simulink model "AUV_Model"  (R2019b)
settings: Solver=VariableStepAuto  StartTime=0.0  StopTime=300  FixedStep=0.5  RelTol=1e-3
InitFcn:
  | mdlWks = get_param(gcs,'ModelWorkspace');
  | a = getVariable(mdlWks,'a');
  | b = getVariable(mdlWks,'b');
  | c = getVariable(mdlWks,'c');
StopFcn:
  | figure(2)
  | plot3(Position_Data(1,1),Position_Data(1,2),Position_Data(1,3),'r*')
  | hold on
  | plot3(Position_Data(:,1),Position_Data(:,2),Position_Data(:,3));
  | plot3(Position_Data(end,1),Position_Data(end,2),Position_Data(end,3),'g*');
  | grid on
  | legend('Start Point','Trajectory','End Point')
model workspace (MAT data in the model file):
  a = 1
  b = 1
  c = 1
undefined symbols (not defined in the file or in its folder): sigbuilder_block
libraries: simulink x6, sharedtransform x6, vrlib x6, dspfdesign x6, shared6dof x1, aerolibasang x1, aerolibnav x1
(part 3 of 3)

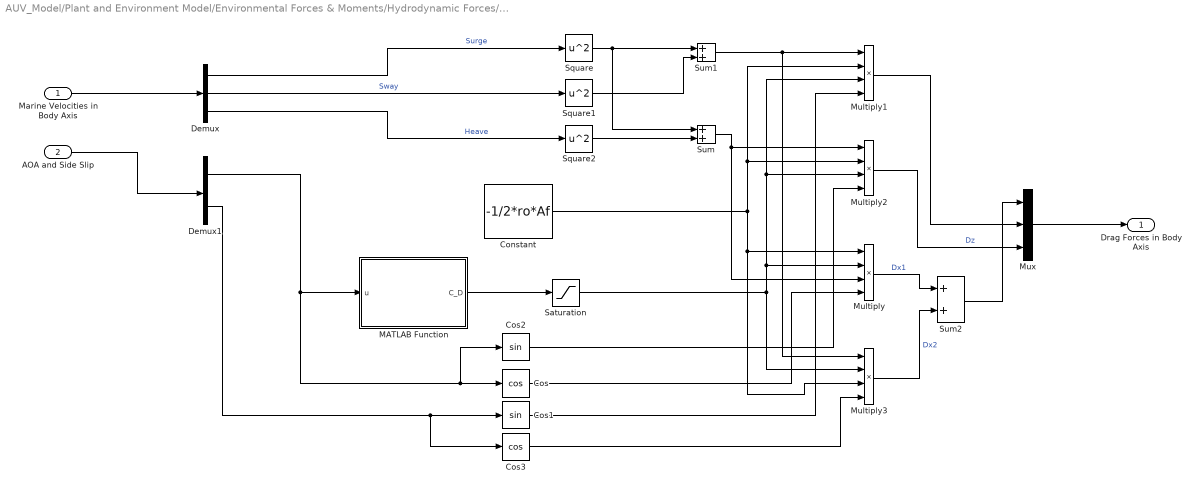
== system AUV_Model/Plant and Environment Model/Environmental Forces & Moments/Hydrodynamic Forces/Hydrodynamic Forces - Accurate/Force Exerted due to Drag (Body Axis) ==
  Marine Velocities in Body Axis : Inport
  AOA and Side Slip : Inport  Port=2
  Constant : Constant  Value=-1/2*ro*Af  mask{ro=1000, Af=0.001}
      mask prompts: ro "Density of Water"; Af "Submarine Frontal Area"
      mask DialogControl DescGroupVar Prompt: Input
      mask DialogControl DescTextVar Prompt: Enter the following values :
  Cos : Trigonometry  Operator=cos
  Cos1 : Trigonometry
  Cos2 : Trigonometry
  Cos3 : Trigonometry  Operator=cos
  Demux : Demux  Outputs=3
  Demux1 : Demux  Outputs=2
  MATLAB Function : MATLAB Function  TreatAsAtomicUnit=on
  Multiply{,1..3} (4 alike) : Product  Inputs=4
  Mux : Mux  Inputs=3
  Saturation : Saturate  UpperLimit=25  LowerLimit=-25
  Square : Math  Operator=square  SaturateOnIntegerOverflow=on
  Square1 : Math  Operator=square  SaturateOnIntegerOverflow=on
  Square2 : Math  Operator=square  SaturateOnIntegerOverflow=on
  Sum : Sum
  Sum1 : Sum
  Sum2 : Sum
  Drag Forces in Body Axis : Outport  VectorParamsAs1DForOutWhenUnconnected=off
  wires:
  Saturation/1 -> Multiply/2, Multiply2/3, Multiply1/3, Multiply3/2
  Square1/1 -> Sum1/2
  Multiply1/1 -> Mux/2
  Sum2/1 -> Mux/1
  Cos3/1 -> Multiply3/4
  AOA and Side Slip/1 -> Demux1/1
  Marine Velocities in Body Axis/1 -> Demux/1
  Cos2/1 -> Multiply2/4
  Mux/1 -> Drag Forces in Body Axis/1
  Square2/1 -> Sum/2
  Demux1/2 -> Cos1/1, Cos3/1
  Demux1/1 -> MATLAB Function/1(u), Cos2/1, Cos/1
  MATLAB Function/1(C_D) -> Saturation/1
  Multiply2/1 -> Mux/3  "Dz"
  Cos/1 -> Multiply/4
  Demux/3 -> Square2/1  "Heave"
  Constant/1 -> Multiply2/2, Multiply1/2, Multiply/1, Multiply3/3
  Multiply3/1 -> Sum2/2  "Dx2"
  Sum/1 -> Multiply/3, Multiply2/1
  Demux/1 -> Square/1  "Surge"
  Multiply/1 -> Sum2/1  "Dx1"
  Sum1/1 -> Multiply1/1, Multiply3/1
  Cos1/1 -> Multiply1/4
  Demux/2 -> Square1/1  "Sway"
  Square/1 -> Sum1/1, Sum/1

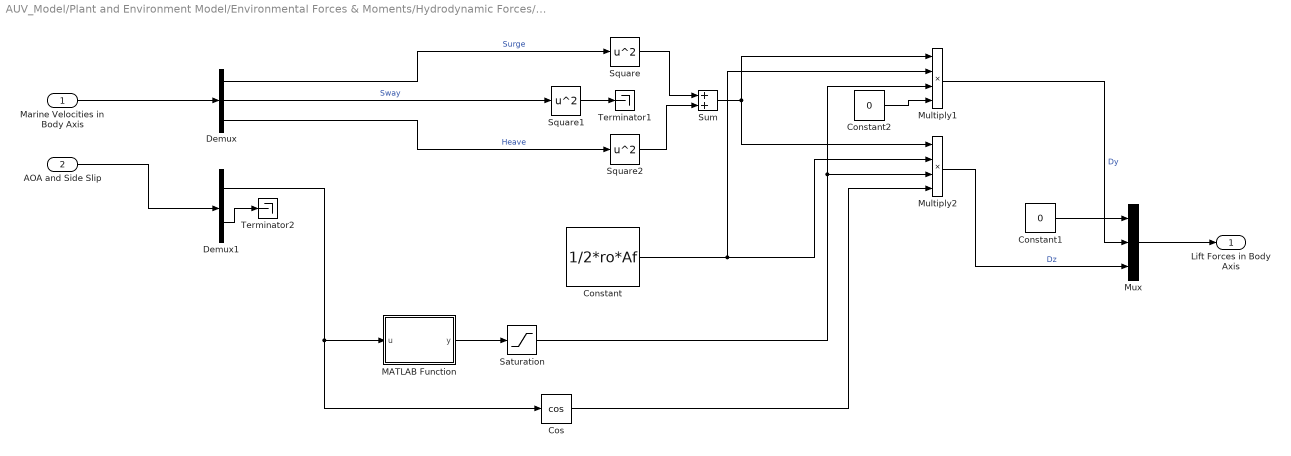
== system AUV_Model/Plant and Environment Model/Environmental Forces & Moments/Hydrodynamic Forces/Hydrodynamic Forces - Accurate/Force Exerted due to Lift (Body Axis) ==
  Marine Velocities in Body Axis : Inport
  AOA and Side Slip : Inport  Port=2
  Constant : Constant  Value=1/2*ro*Af  mask{ro=1000, Af=0.001}
      mask prompts: ro "Density of Water"; Af "Submarine Frontal Area"
      mask DialogControl DescGroupVar Prompt: Input
      mask DialogControl DescTextVar Prompt: Enter the following values :
  Constant1 : Constant  Value=0
  Constant2 : Constant  Value=0
  Cos : Trigonometry  Operator=cos
  Demux : Demux  Outputs=3
  Demux1 : Demux  Outputs=2
  MATLAB Function : MATLAB Function  TreatAsAtomicUnit=on
  Multiply1 : Product  Inputs=4
  Multiply2 : Product  Inputs=4
  Mux : Mux  Inputs=3
  Saturation : Saturate  UpperLimit=25  LowerLimit=-25
  Square : Math  Operator=square  SaturateOnIntegerOverflow=on
  Square1 : Math  Operator=square  SaturateOnIntegerOverflow=on
  Square2 : Math  Operator=square  SaturateOnIntegerOverflow=on
  Sum : Sum
  Terminator1 : Terminator
  Terminator2 : Terminator
  Lift Forces in Body Axis : Outport  VectorParamsAs1DForOutWhenUnconnected=off
  wires:
  Saturation/1 -> Multiply2/3, Multiply1/3
  Constant2/1 -> Multiply1/4
  Multiply2/1 -> Mux/3  "Dz"
  Constant1/1 -> Mux/1
  Cos/1 -> Multiply2/4
  Square/1 -> Sum/1
  Demux/2 -> Square1/1  "Sway"
  Demux/1 -> Square/1  "Surge"
  Sum/1 -> Multiply1/1, Multiply2/1
  Constant/1 -> Multiply1/2, Multiply2/2
  Multiply1/1 -> Mux/2  "Dy"
  Demux/3 -> Square2/1  "Heave"
  MATLAB Function/1(y) -> Saturation/1
  Demux1/1 -> MATLAB Function/1(u), Cos/1
  Square2/1 -> Sum/2
  Mux/1 -> Lift Forces in Body Axis/1
  Marine Velocities in Body Axis/1 -> Demux/1
  AOA and Side Slip/1 -> Demux1/1
  Square1/1 -> Terminator1/1
  Demux1/2 -> Terminator2/1

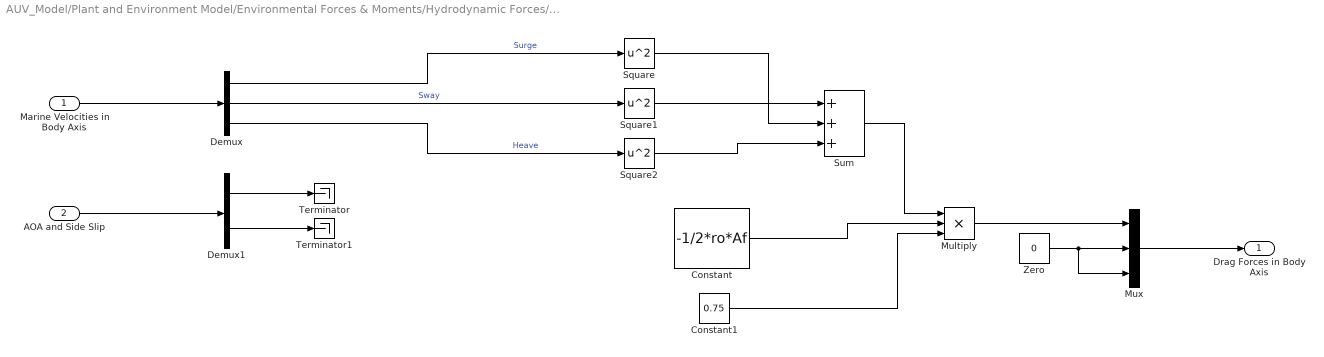
== system AUV_Model/Plant and Environment Model/Environmental Forces & Moments/Hydrodynamic Forces/Hydrodynamic Forces - Basic/Force Exerted due to Drag (Body Axis) ==
  Marine Velocities in Body Axis : Inport
  AOA and Side Slip : Inport  Port=2
  Constant : Constant  Value=-1/2*ro*Af  mask{ro=1000, Af=0.001}
      mask prompts: ro "Density of Water"; Af "Submarine Frontal Area"
      mask DialogControl DescGroupVar Prompt: Input
      mask DialogControl DescTextVar Prompt: Enter the following values :
  Constant1 : Constant  Value=0.75
  Demux : Demux  Outputs=3
  Demux1 : Demux  Outputs=2
  Multiply : Product  Inputs=3
  Mux : Mux  Inputs=3
  Square : Math  Operator=square  SaturateOnIntegerOverflow=on
  Square1 : Math  Operator=square  SaturateOnIntegerOverflow=on
  Square2 : Math  Operator=square  SaturateOnIntegerOverflow=on
  Sum : Sum  Inputs=+++
  Terminator : Terminator
  Terminator1 : Terminator
  Zero : Constant  Value=0  OutDataTypeStr=Inherit: Inherit via back propagation
  Drag Forces in Body Axis : Outport  VectorParamsAs1DForOutWhenUnconnected=off
  wires:
  AOA and Side Slip/1 -> Demux1/1
  Marine Velocities in Body Axis/1 -> Demux/1
  Mux/1 -> Drag Forces in Body Axis/1
  Square2/1 -> Sum/3
  Demux/3 -> Square2/1  "Heave"
  Sum/1 -> Multiply/1
  Demux/1 -> Square/1  "Surge"
  Demux/2 -> Square1/1  "Sway"
  Square/1 -> Sum/2
  Square1/1 -> Sum/1
  Demux1/1 -> Terminator/1
  Demux1/2 -> Terminator1/1
  Constant/1 -> Multiply/2
  Constant1/1 -> Multiply/3
  Multiply/1 -> Mux/1
  Zero/1 -> Mux/3, Mux/2

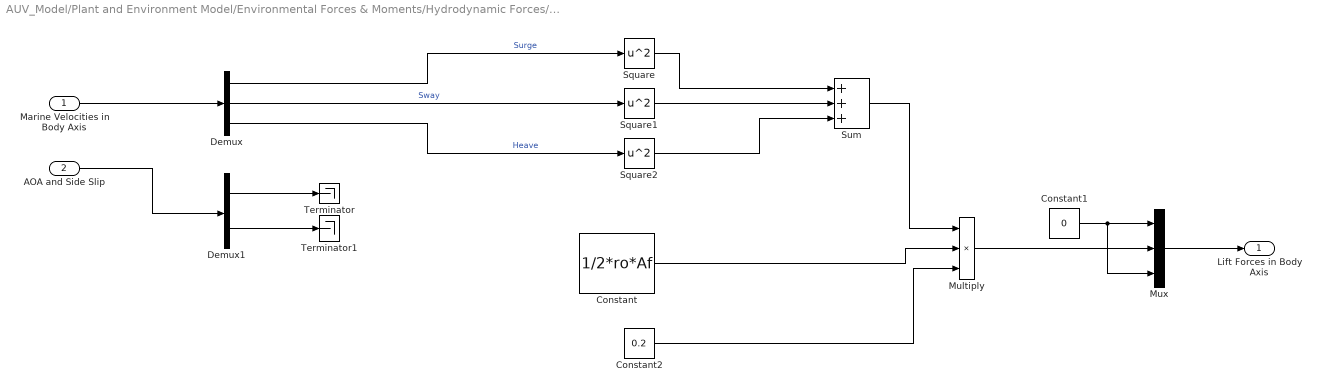
== system AUV_Model/Plant and Environment Model/Environmental Forces & Moments/Hydrodynamic Forces/Hydrodynamic Forces - Basic/Force Exerted due to Lift (Body Axis) ==
  Marine Velocities in Body Axis : Inport
  AOA and Side Slip : Inport  Port=2
  Constant : Constant  Value=1/2*ro*Af  mask{ro=1000, Af=0.001}
      mask prompts: ro "Density of Water"; Af "Submarine Frontal Area"
      mask DialogControl DescGroupVar Prompt: Input
      mask DialogControl DescTextVar Prompt: Enter the following values :
  Constant1 : Constant  Value=0
  Constant2 : Constant  Value=0.2
  Demux : Demux  Outputs=3
  Demux1 : Demux  Outputs=2
  Multiply : Product  Inputs=3
  Mux : Mux  Inputs=3
  Square : Math  Operator=square  SaturateOnIntegerOverflow=on
  Square1 : Math  Operator=square  SaturateOnIntegerOverflow=on
  Square2 : Math  Operator=square  SaturateOnIntegerOverflow=on
  Sum : Sum  Inputs=+++
  Terminator : Terminator
  Terminator1 : Terminator
  Lift Forces in Body Axis : Outport  VectorParamsAs1DForOutWhenUnconnected=off
  wires:
  Constant1/1 -> Mux/3, Mux/1
  Square/1 -> Sum/1
  Demux/2 -> Square1/1  "Sway"
  Demux/1 -> Square/1  "Surge"
  Demux/3 -> Square2/1  "Heave"
  Square2/1 -> Sum/3
  Mux/1 -> Lift Forces in Body Axis/1
  Marine Velocities in Body Axis/1 -> Demux/1
  AOA and Side Slip/1 -> Demux1/1
  Square1/1 -> Sum/2
  Sum/1 -> Multiply/1
  Constant/1 -> Multiply/2
  Constant2/1 -> Multiply/3
  Multiply/1 -> Mux/2
  Demux1/1 -> Terminator/1
  Demux1/2 -> Terminator1/1

== system AUV_Model/Plant and Environment Model/Environmental Forces & Moments/Hydrostatic Forces/Environment Model/3D Rotate Drag ==
  Force : Inport
  "Roll, Pitch, Yaw" : Inport  Port=2
  Gain : Gain
  Matrix Multiply : Product  Multiplication=Matrix(*)
  Rotation Angles to Direction Cosine Matrix : sharedtransform/Rotation Angles to Direction Cosine Matrix  rotationOrder=XYZ  aMode=aMode
      settings: SourceProductBaseCode=AE
  Transpose : Math  Operator=transpose  SaturateOnIntegerOverflow=on
  "Transformed_Force " : Outport  VectorParamsAs1DForOutWhenUnconnected=off
  wires:
  Matrix Multiply/1 -> "Transformed_Force "/1
  Rotation Angles to Direction Cosine Matrix/1 -> Transpose/1
  Force/1 -> Matrix Multiply/2
  "Roll, Pitch, Yaw"/1 -> Gain/1
  Transpose/1 -> Matrix Multiply/1
  Gain/1 -> Rotation Angles to Direction Cosine Matrix/1

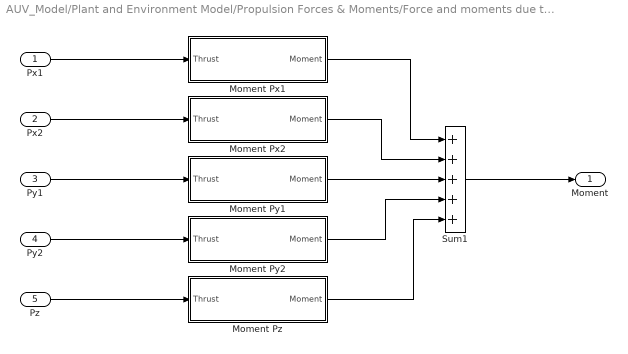
== system AUV_Model/Plant and Environment Model/Propulsion Forces & Moments/Force and moments due to Thrust/Thrust to Propulsion /Moment computation ==
  Px1 : Inport
  Px2 : Inport  Port=2
  Py1 : Inport  Port=3
  Py2 : Inport  Port=4
  Pz : Inport  Port=5
  Moment Px1 : Subsystem  mask{a=0, b=-0.2, c=0}
      mask prompts: a "X Coordinate of Thruster from Center of Buoyancy"; b "Y Coordinate of Thruster from Center of Buoyancy"; c "Z Coordinate of Thruster from Center of Buoyancy"
      mask DialogControl DescTextVar Prompt: Enter Thruster Position w.r.t Center of Buoyancy
  Moment Px2 : Subsystem  mask{a=0, b=0.2, c=0}
      mask prompts: a "X Coordinate of Thruster from Center of Buoyancy"; b "Y Coordinate of Thruster from Center of Buoyancy"; c "Z Coordinate of Thruster from Center of Buoyancy"
      mask DialogControl DescTextVar Prompt: Enter Thruster Position w.r.t Center of Buoyancy
  Moment Py1 : Subsystem  mask{a=.2, b=0, c=0}
      mask prompts: a "X Coordinate of Thruster from Center of Buoyancy"; b "Y Coordinate of Thruster from Center of Buoyancy"; c "Z Coordinate of Thruster from Center of Buoyancy"
      mask DialogControl DescTextVar Prompt: Enter Thruster Position w.r.t Center of Buoyancy
  Moment Py2 : Subsystem  mask{a=-0.2, b=0, c=0}
      mask prompts: a "X Coordinate of Thruster from Center of Buoyancy"; b "Y Coordinate of Thruster from Center of Buoyancy"; c "Z Coordinate of Thruster from Center of Buoyancy"
      mask DialogControl DescTextVar Prompt: Enter Thruster Position w.r.t Center of Buoyancy
  Moment Pz : Subsystem  mask{a=0, b=0, c=0}
      mask prompts: a "X Coordinate of Thruster from Center of Buoyancy"; b "Y Coordinate of Thruster from Center of Buoyancy"; c "Z Coordinate of Thruster from Center of Buoyancy"
      mask DialogControl DescTextVar Prompt: Enter Thruster Position w.r.t Center of Buoyancy
  Sum1 : Sum  Inputs=+++++
  Moment : Outport  VectorParamsAs1DForOutWhenUnconnected=off
  wires:
  Py2/1 -> Moment Py2/1(Thrust)
  Px1/1 -> Moment Px1/1(Thrust)
  Py1/1 -> Moment Py1/1(Thrust)
  Moment Px1/1(Moment) -> Sum1/1
  Moment Px2/1(Moment) -> Sum1/2
  Moment Pz/1(Moment) -> Sum1/5
  Moment Py2/1(Moment) -> Sum1/4
  Pz/1 -> Moment Pz/1(Thrust)
  Moment Py1/1(Moment) -> Sum1/3
  Sum1/1 -> Moment/1
  Px2/1 -> Moment Px2/1(Thrust)

== system AUV_Model/Plant and Environment Model/Propulsion Forces & Moments/Force and moments due to Thrust/Thrust to Propulsion /Thrust Transformation ==
  Thrust Inputs : Inport
  Demux1 : Demux  Outputs=5
  Thrust Px1 : Outport  VectorParamsAs1DForOutWhenUnconnected=off
  Thrust Px2 : Outport  Port=2  VectorParamsAs1DForOutWhenUnconnected=off
  Thrust Py1 : Outport  Port=3  VectorParamsAs1DForOutWhenUnconnected=off
  Thrust Py2 : Outport  Port=4  VectorParamsAs1DForOutWhenUnconnected=off
  Thrust Pz : Outport  Port=5  VectorParamsAs1DForOutWhenUnconnected=off
  wires:
  Demux1/4 -> Thrust Py2/1
  Demux1/5 -> Thrust Pz/1
  Thrust Inputs/1 -> Demux1/1
  Demux1/1 -> Thrust Px1/1
  Demux1/2 -> Thrust Px2/1
  Demux1/3 -> Thrust Py1/1

== system AUV_Model/Plant and Environment Model/Propulsion Forces & Moments/Input commands to Thrust/PWM Signals to Thrust /Thrust_direction Py1 ==
  Thrust : Inport
  Constant : Constant  Value=0
  Constant1 : Constant  Value=0
  Constant2 : Constant  Value=pi/2
  Matrix Multiply : Product  Multiplication=Matrix(*)
  Mux : Mux  Inputs=3
  Rotation Angles to Direction Cosine Matrix : sharedtransform/Rotation Angles to Direction Cosine Matrix  rotationOrder=XYZ  aMode=aMode
      settings: SourceProductBaseCode=AE
  Transpose : Math  Operator=transpose  SaturateOnIntegerOverflow=on
  "Transformed_Thrust " : Outport  VectorParamsAs1DForOutWhenUnconnected=off
  wires:
  Matrix Multiply/1 -> "Transformed_Thrust "/1
  Mux/1 -> Rotation Angles to Direction Cosine Matrix/1
  Rotation Angles to Direction Cosine Matrix/1 -> Transpose/1
  Constant1/1 -> Mux/2
  Thrust/1 -> Matrix Multiply/2
  Constant/1 -> Mux/1
  Transpose/1 -> Matrix Multiply/1
  Constant2/1 -> Mux/3

== system AUV_Model/Plant and Environment Model/Propulsion Forces & Moments/Input commands to Thrust/PWM Signals to Thrust /Thrust_direction Py2 ==
  Thrust : Inport
  Constant : Constant  Value=0
  Constant1 : Constant  Value=0
  Constant2 : Constant  Value=pi/2
  Matrix Multiply : Product  Multiplication=Matrix(*)
  Mux : Mux  Inputs=3
  Rotation Angles to Direction Cosine Matrix : sharedtransform/Rotation Angles to Direction Cosine Matrix  rotationOrder=XYZ  aMode=aMode
      settings: SourceProductBaseCode=AE
  Transpose : Math  Operator=transpose  SaturateOnIntegerOverflow=on
  "Transformed_Thrust " : Outport  VectorParamsAs1DForOutWhenUnconnected=off
  wires:
  Matrix Multiply/1 -> "Transformed_Thrust "/1
  Mux/1 -> Rotation Angles to Direction Cosine Matrix/1
  Rotation Angles to Direction Cosine Matrix/1 -> Transpose/1
  Constant1/1 -> Mux/2
  Thrust/1 -> Matrix Multiply/2
  Constant/1 -> Mux/1
  Transpose/1 -> Matrix Multiply/1
  Constant2/1 -> Mux/3

== system AUV_Model/Plant and Environment Model/Propulsion Forces & Moments/Input commands to Thrust/PWM Signals to Thrust /Thrust_direction Pz ==
  Thrust : Inport
  Constant : Constant  Value=0
  Constant1 : Constant  Value=pi/2
  Constant2 : Constant  Value=0
  Matrix Multiply : Product  Multiplication=Matrix(*)
  Mux : Mux  Inputs=3
  Rotation Angles to Direction Cosine Matrix : sharedtransform/Rotation Angles to Direction Cosine Matrix  rotationOrder=ZYX  aMode=aMode
      settings: SourceProductBaseCode=AE
  Transpose : Math  Operator=transpose  SaturateOnIntegerOverflow=on
  "Transformed_Thrust " : Outport  VectorParamsAs1DForOutWhenUnconnected=off
  wires:
  Matrix Multiply/1 -> "Transformed_Thrust "/1
  Mux/1 -> Rotation Angles to Direction Cosine Matrix/1
  Rotation Angles to Direction Cosine Matrix/1 -> Transpose/1
  Constant1/1 -> Mux/2
  Thrust/1 -> Matrix Multiply/2
  Constant/1 -> Mux/1
  Transpose/1 -> Matrix Multiply/1
  Constant2/1 -> Mux/3

== system AUV_Model/Plant and Environment Model/Propulsion Forces & Moments/Force and moments due to Thrust/Thrust to Propulsion /Moment computation/Moment Px1 ==
  Thrust : Inport
  Constant : Constant  Value=[a;b;c]
  Cross Product : vrlib/Utilities/Cross Product
      settings: SourceProductBaseCode=VR
  Moment : Outport  VectorParamsAs1DForOutWhenUnconnected=off
  wires:
  Cross Product/1 -> Moment/1
  Thrust/1 -> Cross Product/2
  Constant/1 -> Cross Product/1

== system AUV_Model/Plant and Environment Model/Propulsion Forces & Moments/Force and moments due to Thrust/Thrust to Propulsion /Moment computation/Moment Px2 ==
  Thrust : Inport
  Constant : Constant  Value=[a;b;c]
  Cross Product : vrlib/Utilities/Cross Product
      settings: SourceProductBaseCode=VR
  Moment : Outport  VectorParamsAs1DForOutWhenUnconnected=off
  wires:
  Constant/1 -> Cross Product/1
  Thrust/1 -> Cross Product/2
  Cross Product/1 -> Moment/1

== system AUV_Model/Plant and Environment Model/Propulsion Forces & Moments/Force and moments due to Thrust/Thrust to Propulsion /Moment computation/Moment Py1 ==
  Thrust : Inport
  Constant : Constant  Value=[a;b;c]
  Cross Product : vrlib/Utilities/Cross Product
      settings: SourceProductBaseCode=VR
  Moment : Outport  VectorParamsAs1DForOutWhenUnconnected=off
  wires:
  Cross Product/1 -> Moment/1
  Thrust/1 -> Cross Product/2
  Constant/1 -> Cross Product/1

== system AUV_Model/Plant and Environment Model/Propulsion Forces & Moments/Force and moments due to Thrust/Thrust to Propulsion /Moment computation/Moment Py2 ==
  Thrust : Inport
  Constant : Constant  Value=[a;b;c]
  Cross Product : vrlib/Utilities/Cross Product
      settings: SourceProductBaseCode=VR
  Moment : Outport  VectorParamsAs1DForOutWhenUnconnected=off
  wires:
  Constant/1 -> Cross Product/1
  Thrust/1 -> Cross Product/2
  Cross Product/1 -> Moment/1

== system AUV_Model/Plant and Environment Model/Propulsion Forces & Moments/Force and moments due to Thrust/Thrust to Propulsion /Moment computation/Moment Pz ==
  Thrust : Inport
  Constant : Constant  Value=[a;b;c]
  Cross Product : vrlib/Utilities/Cross Product
      settings: SourceProductBaseCode=VR
  Moment : Outport  VectorParamsAs1DForOutWhenUnconnected=off
  wires:
  Cross Product/1 -> Moment/1
  Thrust/1 -> Cross Product/2
  Constant/1 -> Cross Product/1

== matlab function AUV_Model/Plant and Environment Model/Environmental Forces & Moments/Hydrodynamic Forces/Hydrodynamic Forces - Accurate/Force Exerted due to Drag (Body Axis)/MATLAB Function ==
  data: u input; C_D output
function C_D = Calculate_Drag_Coeff(u)
if u>pi/2
    u = u-pi;
elseif u < -pi/2
    u = u + pi;
end
C_D = 5.25*(u.^2) - 0.315 * (u) + 0.732;

== matlab function AUV_Model/Plant and Environment Model/Environmental Forces & Moments/Hydrodynamic Forces/Hydrodynamic Forces - Accurate/Force Exerted due to Lift (Body Axis)/MATLAB Function ==
  data: u input; y output
function y = fcn(u)
if u>pi/2
    u = u-pi;
elseif u < -pi/2
    u = u + pi;
end

y = 1 * (u) + 0;

== matlab function AUV_Model/Plant and Environment Model/Propulsion Forces & Moments/Input commands to Thrust/PWM Signals to Thrust /MATLAB Function ==
  data: u input; y output
function y = Normalize(u)
y = (u-1500)*150/400;

== matlab function AUV_Model/Plant and Environment Model/Propulsion Forces & Moments/Input commands to Thrust/PWM Signals to Thrust /MATLAB Function1 ==
  data: u input; y output
function y = Normalize(u)
y = (u-1500)*150/400;

== matlab function AUV_Model/Plant and Environment Model/Propulsion Forces & Moments/Input commands to Thrust/PWM Signals to Thrust /MATLAB Function2 ==
  data: u input; y output
function y = Normalize(u)
y = (u-1500)*150/400;

== matlab function AUV_Model/Plant and Environment Model/Propulsion Forces & Moments/Input commands to Thrust/PWM Signals to Thrust /MATLAB Function3 ==
  data: u input; y output
function y = Normalize(u)
y = (u-1500)*150/400;

== matlab function AUV_Model/Plant and Environment Model/Propulsion Forces & Moments/Input commands to Thrust/PWM Signals to Thrust /MATLAB Function4 ==
  data: u input; y output
function y = Normalize(u)
y = (u-1500)*150/400;

== matlab function AUV_Model/Plant and Environment Model/Dynamics solver/Post-Processing/MATLAB Function ==
  data: Position input; srf_in input
function Visualize(Position, srf_in)

    coder.extrinsic('setax'); 
    setax(Position, srf_in);  

end
